simulink library "AEMACE10_IN"  (R2021b)
settings: Solver=VariableStepAuto  StartTime=0.0  StopTime=10.0  RelTol=1e-3
values from neighbouring files (symbols this model uses):
  dataAEMACE = 60.0    [applicationDD.sldd]    (also in dataAEMACE.mat = ; dataAEMACE_DD.sldd)
settings Model: Creator=ACH  LastModifiedBy=ACH

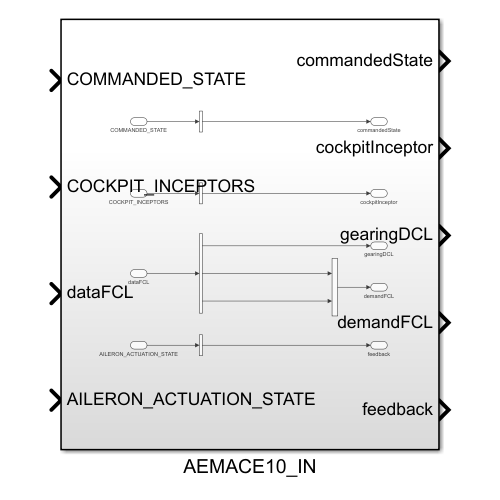
[thumbnail: Simulink's stored preview of the top-level diagram]
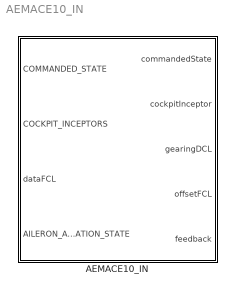
== system AEMACE10_IN ==
  AEMACE10_IN : Subsystem

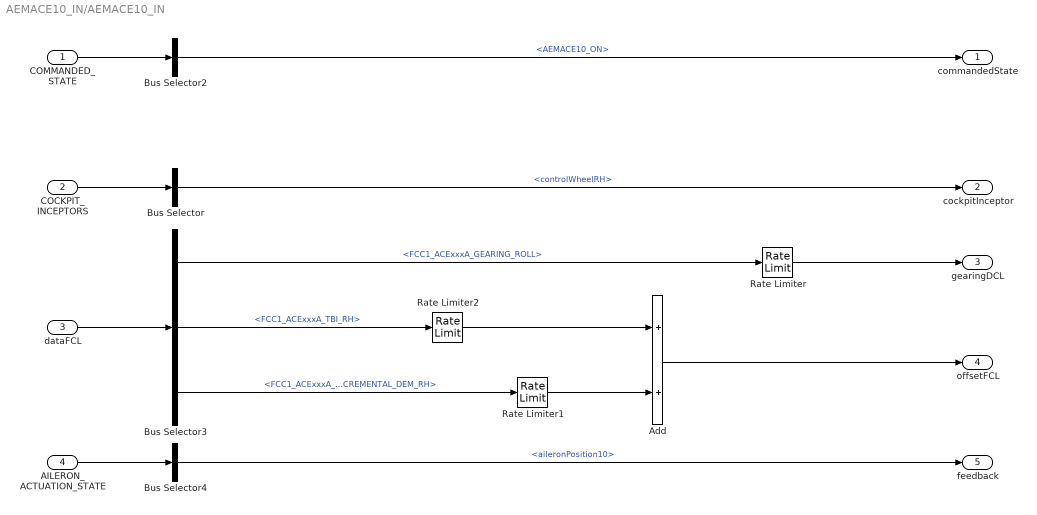
== system AEMACE10_IN/AEMACE10_IN ==
  COMMANDED_STATE : Inport  OutDataTypeStr=Bus: COMMANDED_STATE
  COCKPIT_INCEPTORS : Inport  Port=2  OutDataTypeStr=Bus: COCKPIT_INCEPTORS
  dataFCL : Inport  Port=3  OutDataTypeStr=Bus: FCC1_ACExxxA_C1_A
  AILERON_ACTUATION_STATE : Inport  Port=4  OutDataTypeStr=Bus: AILERON_ACTUATION_STATE
  Add : Sum
  Bus Selector : BusSelector  OutputSignals=controlWheelRH
  Bus Selector2 : BusSelector  OutputSignals=AEMACE10_ON
  Bus Selector3 : BusSelector  OutputSignals=FCC1_ACExxxA_GEARING_ROLL,FCC1_ACExxxA_TBI_RH,FCC1_ACExxxA_ROLL_INCREMENTAL_DEM_RH
  Bus Selector4 : BusSelector  OutputSignals=aileronPosition10
  Rate Limiter : RateLimiter  RisingSlewLimit=dataAEMACE.rateLimiterGearing  FallingSlewLimit=-dataAEMACE.rateLimiterGearing  SampleTimeMode=inherited
      settings: AttributesFormatString=|
      | %<RisingSlewLimit>
      | %<FallingSlewLimit>
  Rate Limiter1 : RateLimiter  RisingSlewLimit=dataAEMACE.rateLimiterIncrementalDemand  FallingSlewLimit=-dataAEMACE.rateLimiterIncrementalDemand  SampleTimeMode=inherited
      settings: AttributesFormatString=|
      | %<RisingSlewLimit>
      | %<FallingSlewLimit>
  Rate Limiter2 : RateLimiter  RisingSlewLimit=dataAEMACE.rateLimiterTBI  FallingSlewLimit=-dataAEMACE.rateLimiterTBI  SampleTimeMode=inherited
      settings: AttributesFormatString=|
      | %<RisingSlewLimit>
      | %<FallingSlewLimit>
  commandedState : Outport
  cockpitInceptor : Outport  Port=2
  gearingDCL : Outport  Port=3
  offsetFCL : Outport  Port=4
  feedback : Outport  Port=5
  wires:
  Bus Selector3/3 -> Rate Limiter1/1  "<FCC1_ACExxxA_ROLL_INCREMENTAL_DEM_RH>"
  Add/1 -> offsetFCL/1
  Bus Selector3/2 -> Rate Limiter2/1  "<FCC1_ACExxxA_TBI_RH>"
  AILERON_ACTUATION_STATE/1 -> Bus Selector4/1
  Bus Selector2/1 -> commandedState/1  "<AEMACE10_ON>"
  Bus Selector4/1 -> feedback/1  "<aileronPosition10>"
  COMMANDED_STATE/1 -> Bus Selector2/1
  dataFCL/1 -> Bus Selector3/1
  COCKPIT_INCEPTORS/1 -> Bus Selector/1
  Bus Selector/1 -> cockpitInceptor/1  "<controlWheelRH>"
  Bus Selector3/1 -> Rate Limiter/1  "<FCC1_ACExxxA_GEARING_ROLL>"
  Rate Limiter2/1 -> Add/1
  Rate Limiter1/1 -> Add/2
  Rate Limiter/1 -> gearingDCL/1
